simulink model "Lab05"  (R2021b)
settings: Solver=VariableStepAuto  StartTime=0.0  StopTime=10.0  RelTol=1e-3
values from neighbouring files (symbols this model uses):
  A0 = eye(3)    [Lab05_script.m]
  h_N_target = h_0_N    [Lab05_script.m]
  I = [Ix 0 0; 0 Iy 0; 0 0 Iz]    [Lab05_script.m]
  I_inv = inv(I)    [Lab05_script.m]
  v1 = [0 1 -1]'    [Lab05_script.m]
  v2 = [-1 0 1]'    [Lab05_script.m]
  v3 = [1 -1 0]'    [Lab05_script.m]
  w_0 = [wx_0; wy_0; wz_0]    [Lab05_script.m]
libraries: matrix_library x1
settings Model: Creator=samuz  LastModifiedBy=samuz

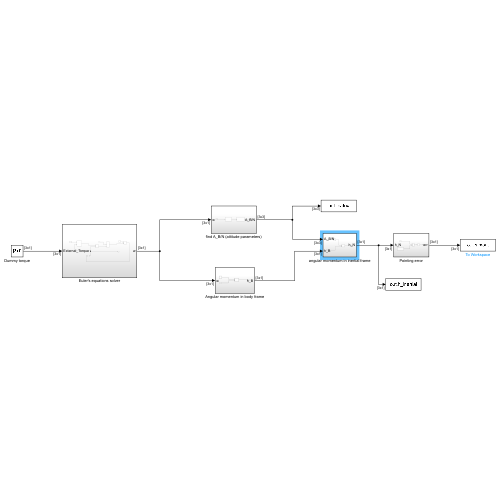
[thumbnail: Simulink's stored preview of the top-level diagram]
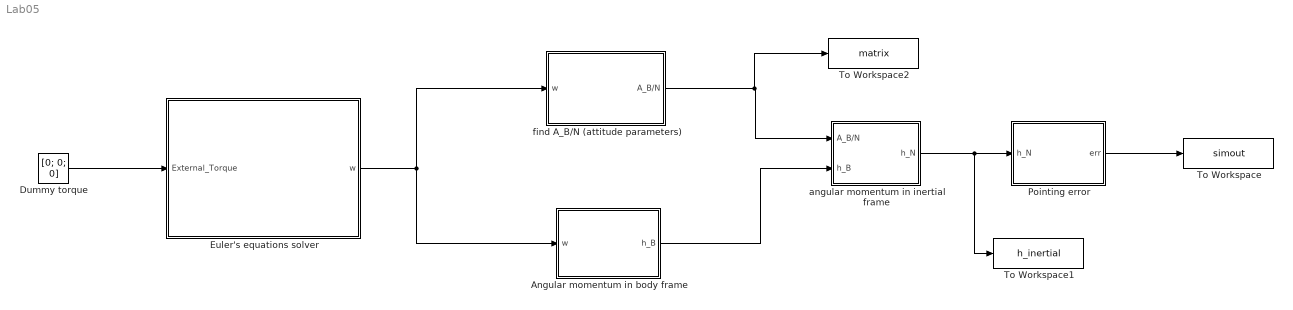
== system Lab05 ==
  Angular momentum in body frame : Subsystem
  Dummy torque : Constant  Value=[0; 0; 0]  VectorParams1D=off
  Euler's equations solver : Subsystem
  Pointing error : Subsystem
  To Workspace : ToWorkspace  VariableName=simout  SampleTime=-1
  To Workspace1 : ToWorkspace  VariableName=h_inertial  SampleTime=-1
  To Workspace2 : ToWorkspace  VariableName=matrix  SampleTime=-1
  angular momentum in inertial frame : Subsystem
  find A_B/N (attitude parameters) : Subsystem
  wires:
  Dummy torque/1 -> Euler's equations solver/1(External_Torque)
  Euler's equations solver/1(w) -> find A_B/N (attitude parameters)/1(w), Angular momentum in body frame/1(w)
  find A_B/N (attitude parameters)/1(A_B/N) -> To Workspace2/1, angular momentum in inertial frame/1(A_B/N)
  Angular momentum in body frame/1(h_B) -> angular momentum in inertial frame/2(h_B)
  angular momentum in inertial frame/1(h_N) -> To Workspace1/1, Pointing error/1(h_N)
  Pointing error/1(err) -> To Workspace/1

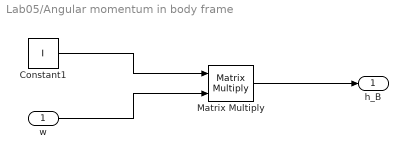
== system Lab05/Angular momentum in body frame ==
  w : Inport
  Constant1 : Constant  Value=I
  Matrix Multiply : Product  Multiplication=Matrix(*)
  h_B : Outport
  wires:
  w/1 -> Matrix Multiply/2
  Matrix Multiply/1 -> h_B/1
  Constant1/1 -> Matrix Multiply/1

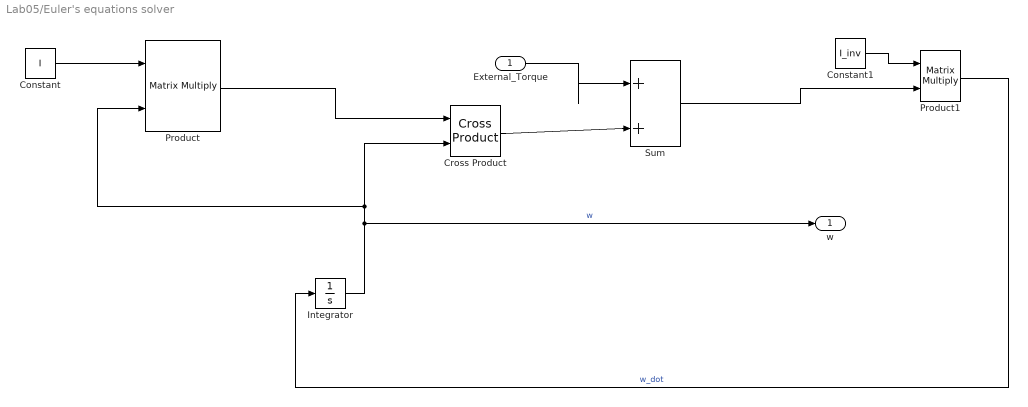
== system Lab05/Euler's equations solver ==
  External_Torque : Inport
  Constant : Constant  Value=I  VectorParams1D=off
  Constant1 : Constant  Value=I_inv  VectorParams1D=off
  Cross Product : matrix_library/Cross Product
      settings: SourceProductBaseCode=SL
  Integrator : Integrator  InitialCondition=w_0
  Product : Product  Multiplication=Matrix(*)
  Product1 : Product  Multiplication=Matrix(*)
  Sum : Sum  Inputs=|++
  w : Outport
  wires:
  Product/1 -> Cross Product/1
  Constant/1 -> Product/1
  Constant1/1 -> Product1/1
  Integrator/1 -> Cross Product/2, Product/2, w/1  "w"
  Product1/1 -> Integrator/1  "w_dot"
  External_Torque/1 -> Sum/1
  Cross Product/1 -> Sum/2
  Sum/1 -> Product1/2

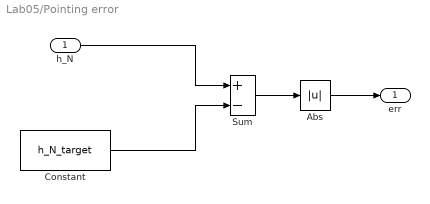
== system Lab05/Pointing error ==
  h_N : Inport
  Abs : Abs
  Constant : Constant  Value=h_N_target  VectorParams1D=off
  Sum : Sum  Inputs=+-
  err : Outport
  wires:
  Constant/1 -> Sum/2
  h_N/1 -> Sum/1
  Sum/1 -> Abs/1
  Abs/1 -> err/1

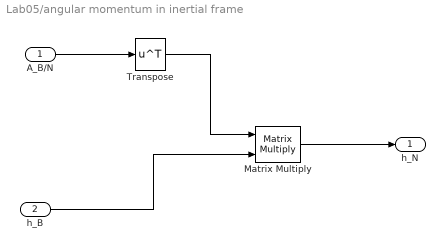
== system Lab05/angular momentum in inertial frame ==
  A_B/N : Inport
  h_B : Inport  Port=2
  Matrix Multiply : Product  Multiplication=Matrix(*)
  Transpose : Math  Operator=transpose  SaturateOnIntegerOverflow=on
  h_N : Outport
  wires:
  Transpose/1 -> Matrix Multiply/1
  Matrix Multiply/1 -> h_N/1
  A_B/N/1 -> Transpose/1
  h_B/1 -> Matrix Multiply/2

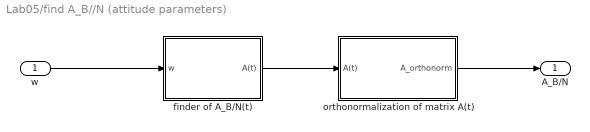
== system Lab05/find A_B//N (attitude parameters) ==
  w : Inport
  finder of A_B/N(t) : Subsystem
  orthonormalization of matrix A(t) : Subsystem
  A_B/N : Outport
  wires:
  w/1 -> finder of A_B/N(t)/1(w)
  finder of A_B/N(t)/1(A(t)) -> orthonormalization of matrix A(t)/1(A(t))
  orthonormalization of matrix A(t)/1(A_orthonorm) -> A_B/N/1

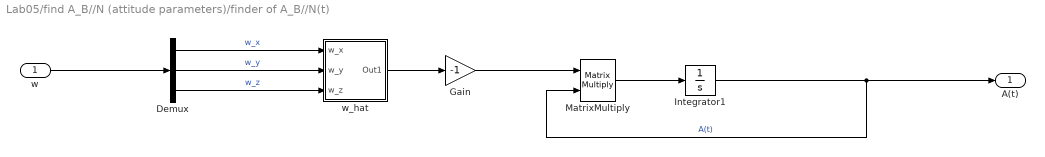
== system Lab05/find A_B//N (attitude parameters)/finder of A_B//N(t) ==
  w : Inport
  Demux : Demux  Outputs=3
  Gain : Gain  Gain=-1
  Integrator1 : Integrator  InitialCondition=A0
  MatrixMultiply : Product  Multiplication=Matrix(*)
  w_hat : Subsystem
  A(t) : Outport
  wires:
  w/1 -> Demux/1
  Gain/1 -> MatrixMultiply/1
  Integrator1/1 -> A(t)/1, MatrixMultiply/2  "A(t)"
  w_hat/1(Out1) -> Gain/1
  Demux/3 -> w_hat/3(w_z)  "w_z"
  Demux/2 -> w_hat/2(w_y)  "w_y"
  Demux/1 -> w_hat/1(w_x)  "w_x"
  MatrixMultiply/1 -> Integrator1/1

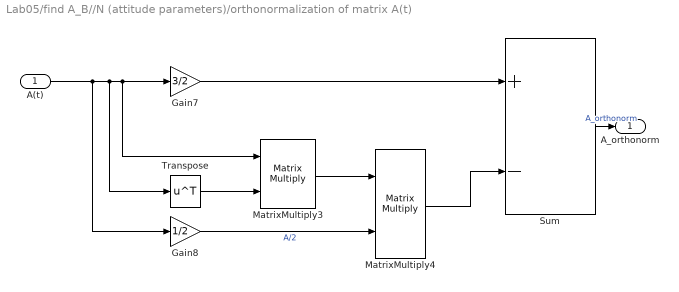
== system Lab05/find A_B//N (attitude parameters)/orthonormalization of matrix A(t) ==
  A(t) : Inport
  Gain7 : Gain  Gain=3/2
  Gain8 : Gain  Gain=1/2
  MatrixMultiply3 : Product  Multiplication=Matrix(*)
  MatrixMultiply4 : Product  Multiplication=Matrix(*)
  Sum : Sum  Inputs=+-
  Transpose : Math  Operator=transpose  SaturateOnIntegerOverflow=on
  A_orthonorm : Outport
  wires:
  Transpose/1 -> MatrixMultiply3/2
  MatrixMultiply4/1 -> Sum/2
  MatrixMultiply3/1 -> MatrixMultiply4/1
  Gain7/1 -> Sum/1
  Gain8/1 -> MatrixMultiply4/2  "A/2"
  A(t)/1 -> Gain8/1, Transpose/1, MatrixMultiply3/1, Gain7/1
  Sum/1 -> A_orthonorm/1  "A_orthonorm"

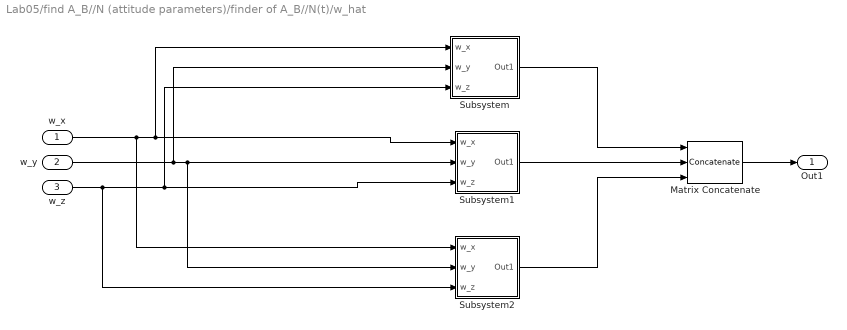
== system Lab05/find A_B//N (attitude parameters)/finder of A_B//N(t)/w_hat ==
  w_x : Inport
  w_y : Inport  Port=2
  w_z : Inport  Port=3
  Matrix Concatenate : Concatenate  NumInputs=3  Mode=Multidimensional array  ConcatenateDimension=2
  Subsystem : Subsystem
  Subsystem1 : Subsystem
  Subsystem2 : Subsystem
  Out1 : Outport
  wires:
  w_y/1 -> Subsystem1/2(w_y), Subsystem2/2(w_y), Subsystem/2(w_y)
  w_z/1 -> Subsystem2/3(w_z), Subsystem/3(w_z), Subsystem1/3(w_z)
  w_x/1 -> Subsystem2/1(w_x), Subsystem/1(w_x), Subsystem1/1(w_x)
  Subsystem2/1(Out1) -> Matrix Concatenate/3
  Subsystem1/1(Out1) -> Matrix Concatenate/2
  Subsystem/1(Out1) -> Matrix Concatenate/1
  Matrix Concatenate/1 -> Out1/1

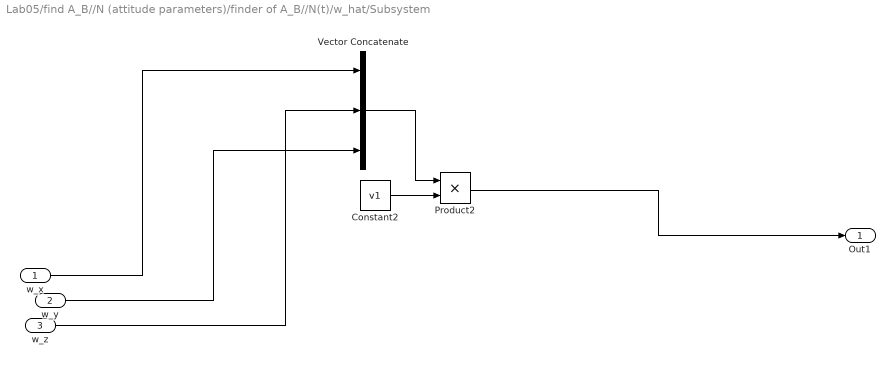
== system Lab05/find A_B//N (attitude parameters)/finder of A_B//N(t)/w_hat/Subsystem ==
  w_x : Inport
  w_y : Inport  Port=2
  w_z : Inport  Port=3
  Constant2 : Constant  Value=v1
  Product2 : Product
  Vector Concatenate : Concatenate  NumInputs=3
  Out1 : Outport
  wires:
  Product2/1 -> Out1/1
  Vector Concatenate/1 -> Product2/1
  Constant2/1 -> Product2/2
  w_x/1 -> Vector Concatenate/1
  w_z/1 -> Vector Concatenate/2
  w_y/1 -> Vector Concatenate/3

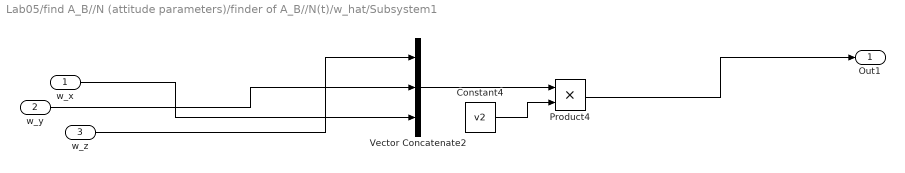
== system Lab05/find A_B//N (attitude parameters)/finder of A_B//N(t)/w_hat/Subsystem1 ==
  w_x : Inport
  w_y : Inport  Port=2
  w_z : Inport  Port=3
  Constant4 : Constant  Value=v2
  Product4 : Product
  Vector Concatenate2 : Concatenate  NumInputs=3
  Out1 : Outport
  wires:
  Constant4/1 -> Product4/2
  Vector Concatenate2/1 -> Product4/1
  Product4/1 -> Out1/1
  w_x/1 -> Vector Concatenate2/3
  w_y/1 -> Vector Concatenate2/2
  w_z/1 -> Vector Concatenate2/1

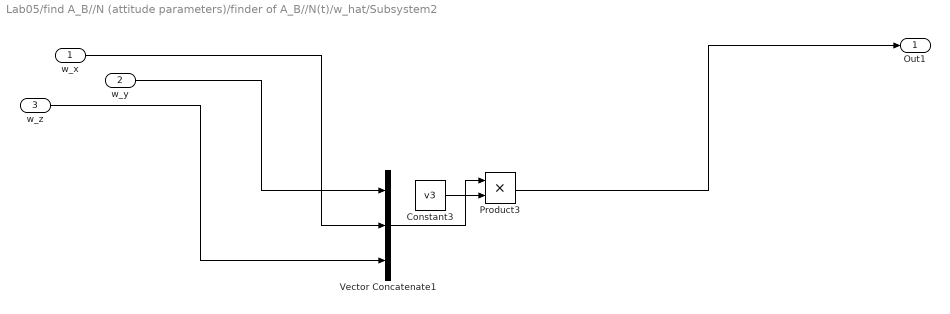
== system Lab05/find A_B//N (attitude parameters)/finder of A_B//N(t)/w_hat/Subsystem2 ==
  w_x : Inport
  w_y : Inport  Port=2
  w_z : Inport  Port=3
  Constant3 : Constant  Value=v3
  Product3 : Product
  Vector Concatenate1 : Concatenate  NumInputs=3
  Out1 : Outport
  wires:
  Product3/1 -> Out1/1
  Constant3/1 -> Product3/2
  w_y/1 -> Vector Concatenate1/1
  Vector Concatenate1/1 -> Product3/1
  w_x/1 -> Vector Concatenate1/2
  w_z/1 -> Vector Concatenate1/3
